simulink model "lab5_es1_sim"  (R2023b)
settings: Solver=VariableStepAuto  StartTime=0.0  StopTime=15  MaxStep=Ts * 0.001  MinStep=Ts * 0.0001  RelTol=1e-3
values from neighbouring files (symbols this model uses):
  C = [1 0]    [lab5_es1.m]
  Kq = Kaug(1)    [lab5_es1.m]
  Kx = Kaug(2:n+1)    [lab5_es1.m]
  Ts = 0.05    [lab5_es1.m]
undefined symbols (not defined in the file or in its folder): DiscIntNeverNeededParam
libraries: cstblocks x1
settings Model: Creator=lucapili  LastModifiedBy=lucapili
settings SolverCC: InitialStep=Ts * 0.0001

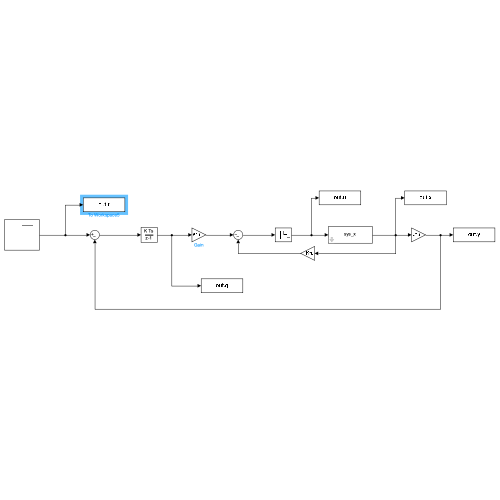
[thumbnail: Simulink's stored preview of the top-level diagram]
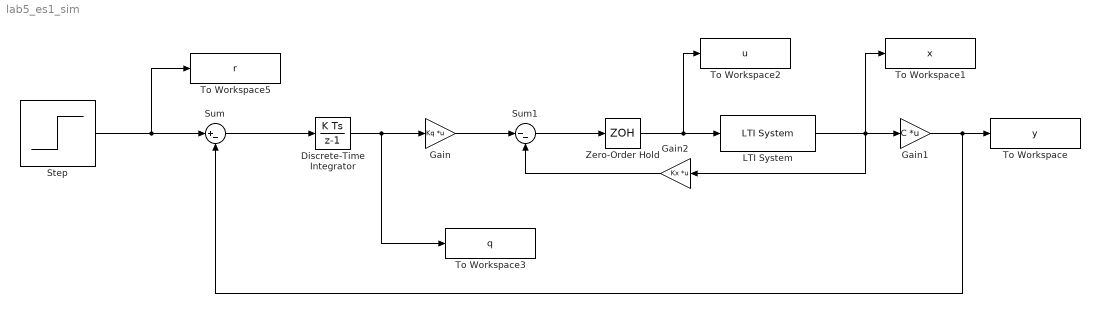
== system lab5_es1_sim ==
  Discrete-Time Integrator : DiscreteIntegrator  SampleTime=-1  ICPrevOutput=DiscIntNeverNeededParam  ICPrevScaledInput=DiscIntNeverNeededParam
  Gain : Gain  Gain=Kq  Multiplication=Matrix(K*u)
  Gain1 : Gain  Gain=C  Multiplication=Matrix(K*u)
  Gain2 : Gain  Gain=Kx  Multiplication=Matrix(K*u)
  LTI System : cstblocks/LTI System  sys=sys_x  IC=x0  PadeOrder=0
  Step : Step  SampleTime=0
  Sum : Sum  Inputs=|+-
  Sum1 : Sum  Inputs=|--
  To Workspace : ToWorkspace  VariableName=y  SaveFormat=Timeseries  SampleTime=Ts*0.001
  To Workspace1 : ToWorkspace  VariableName=x  SaveFormat=Timeseries  SampleTime=Ts*0.001
  To Workspace2 : ToWorkspace  VariableName=u  SaveFormat=Timeseries  SampleTime=Ts * 0.001
  To Workspace3 : ToWorkspace  VariableName=q  SaveFormat=Timeseries  SampleTime=Ts
  To Workspace5 : ToWorkspace  VariableName=r  SaveFormat=Timeseries  SampleTime=Ts*0.001
  Zero-Order Hold : ZeroOrderHold  SampleTime=Ts
  wires:
  Step/1 -> To Workspace5/1, Sum/1
  Sum/1 -> Discrete-Time Integrator/1
  Discrete-Time Integrator/1 -> To Workspace3/1, Gain/1
  Gain/1 -> Sum1/1
  Sum1/1 -> Zero-Order Hold/1
  Zero-Order Hold/1 -> To Workspace2/1, LTI System/1
  LTI System/1 -> Gain2/1, To Workspace1/1, Gain1/1
  Gain1/1 -> Sum/2, To Workspace/1
  Gain2/1 -> Sum1/2
